simulink model "sxem5"  (R2015b)
settings: Solver=VariableStepAuto  StartTime=0.0  StopTime=5  RelTol=1e-3
settings Model: Creator=hohotulca  LastModifiedBy=hohotulca

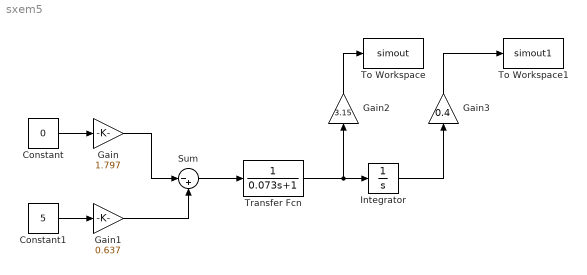
== system sxem5 ==
  Constant : Constant  Value=0
  Constant1 : Constant  Value=5
  Gain : Gain  Gain=1.797
  Gain1 : Gain  Gain=0.637
  Gain2 : Gain  Gain=3.15
  Gain3 : Gain  Gain=0.4
  Integrator : Integrator
  Sum : Sum  Inputs=|-+
  To Workspace : ToWorkspace  VariableName=simout  SaveFormat=Timeseries  SampleTime=-1
  To Workspace1 : ToWorkspace  VariableName=simout1  SaveFormat=Timeseries  SampleTime=-1
  Transfer Fcn : TransferFcn  Denominator=[0.073 1]
  wires:
  Constant/1 -> Gain/1
  Constant1/1 -> Gain1/1
  Gain1/1 -> Sum/2
  Gain/1 -> Sum/1
  Sum/1 -> Transfer Fcn/1
  Transfer Fcn/1 -> Gain2/1, Integrator/1
  Integrator/1 -> Gain3/1
  Gain2/1 -> To Workspace/1
  Gain3/1 -> To Workspace1/1
